simulink model "ControllerIntegration"  (R2020a)
settings: configuration reference "Configuration" (kept outside this file)
undefined symbols (not defined in the file or in its folder): Param
settings Model: Creator=12650014  LastModifiedBy=12650008
settings ConfigSetRef: SourceName=Configuration  SourceLocation=Base Workspace

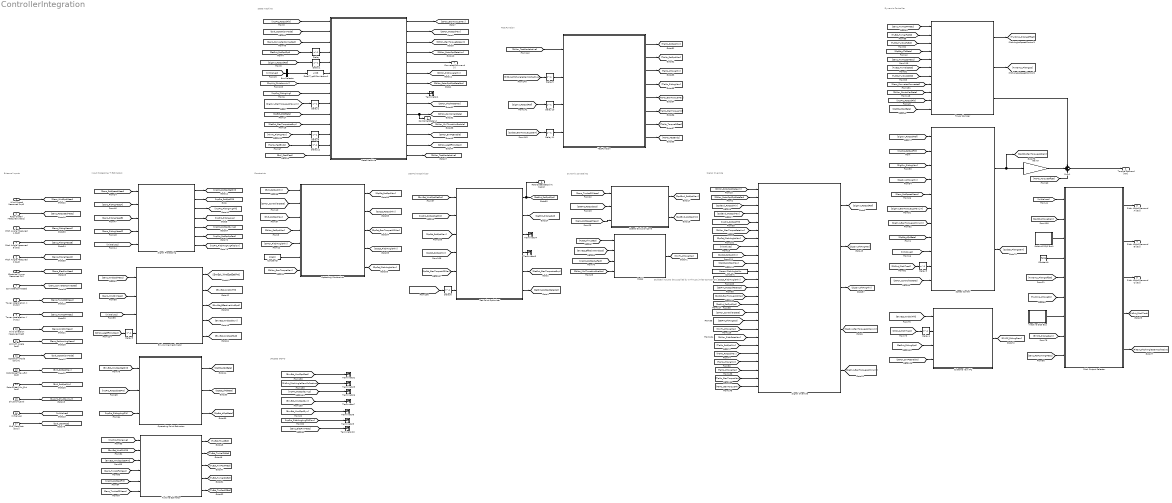
== system ControllerIntegration ==
  note: Stubbed input to be supplied by a Thrust Limiter Component
  note: UNUSED GOTO
  note: Dynamic constraints
  note: Set Point Optimizer
  note: Signal Override
  note: State machine
  note: Constraints
  note: Dynamic Controller
  note: Input Processing + Estimators
  note: External inputs
  note: Test Function
  Wind Speed Measured [m/s] : Inport
  Rotor Speed Measured [rad/s] : Inport  Port=2
  Pitch Angle Measured A [rad] : Inport  Port=3
  Pitch Angle Measured B [rad] : Inport  Port=4
  Pitch Angle Measured C [rad] : Inport  Port=5
  Electrical Power Measured [W] : Inport  Port=6
  ConverterConnected : Inport  Port=7
  Tower Acceleration X [m/s2] : Inport  Port=8
  Tower Acceleration Y [m/s2] : Inport  Port=9
  Wind Direction Measured [rad] : Inport  Port=10
  Azimuth Angle [rad] : Inport  Port=11
  Operation Mode [enum] : Inport  Port=12  OutDataTypeStr=Enum: OpMode
  RotorSpeedMax_Ext [rad] : Inport  Port=13
  RotorSpeedMin_Ext [rad] : Inport  Port=14
  ShudownLevel : Inport  Port=15
  InitValues : Inport  Port=16  OutDataTypeStr=Bus: InitVals
  Extl_StartTest [bool] : Inport  Port=17  OutDataTypeStr=boolean
  Bus Selector : BusSelector  OutputSignals=ControllerState
  Constant : Constant  Value=Param.PitchAngleMin
  Constant1 : Constant  Value=false
  Constant3 : Constant  Value=10e10
  Data Type Conversion1 : DataTypeConversion  OutDataTypeStr=uint8  RndMeth=Round
  Delay{,1..6,8..12} (12 alike) : Delay  DelayLength=1  InitialCondition=0
  Environment estimator : ModelReference  ModelNameDialog=EnvironmentEstimator.slx  SimulationMode=Normal  ModelReferenceVersion=1.228
  Extreme Yaw IPC : ModelReference  ModelNameDialog=ExtremeYawIPC.slx  SimulationMode=Normal  ModelReferenceVersion=1.200
  Gain9 : Gain  Gain=1/Param.GearRatio
  Inactive DQ0 Bus : Subsystem
  Inactive DQ0 Bus1 : Subsystem
  Model : ModelReference  ModelNameDialog=MinimumThrustLimiter.slx  SimulationMode=Normal  ModelReferenceVersion=1.237
  Operating Constraints : ModelReference  ModelNameDialog=OperatingConstraints.slx  SimulationMode=Normal  ModelReferenceVersion=1.199
  Operating Point Estimator : ModelReference  ModelNameDialog=OperatingPointEstimator.slx  SimulationMode=Normal  ModelReferenceVersion=1.187
  Pitch Output Selector : ModelReference  ModelNameDialog=PitchOutputSelector.slx  SimulationMode=Normal  ModelReferenceVersion=1.211
  Set Point Optimizer : ModelReference  ModelNameDialog=SetPointOptimizer.slx  SimulationMode=Normal  ModelReferenceVersion=1.164
  Signal Override : ModelReference  ModelNameDialog=SignalOverride.slx  SimulationMode=Normal  ModelReferenceVersion=1.219
  Signal Processing : ModelReference  ModelNameDialog=SignalProcessing.slx  SimulationMode=Normal  ModelReferenceVersion=1.117
  Speed Control : ModelReference  ModelNameDialog=SpeedController.slx  SimulationMode=Normal  ModelReferenceVersion=1.218
      settings: PortSchema="{\"entries\":[{\"content\":{\"sides\":[{\"content\":{\"connectorIds\":[\"In1\",\"In2\",\"In3\",\"In4\",\"In9\",\"In5\",\"In6\",\"In8\",\"In7\",\"In10\",\"In11\"]},\"type\":\"ConnectorPlacement.EquallySpacedRectSide\",\"uuid\":\"0d9f98d5-5863-4158-b9d8-c1cd92811ae6\"},{\"content\":{\"connectorIds\":[\"Out1\",\"Out2\"],\"side\":\"RIGHT\"},\"type\":\"ConnectorPlacement.EquallySpacedRectSide\",\"uuid\":\"8166d279-4671-4a5d-9b5c-a0ddc413a77e\"},{\"content\":{\"connectorIds\":[],\"side\":\"TOP\"},\"type\":\"ConnectorPlacement.EquallySpacedRectSide\",\"uuid\":\"e681da18-f7d9-4182-9560-dcdd8831121b\"}]},\"type\":\"ConnectorPlacement.EquallySpacedConnector\",\"uuid\":\"20163037-d862-4ea8-8a87-0fce0e65d82b\"}],\"packageUris\":[\"http://schema.mathworks.com/mf0/Connector/19700101\"],\"version\":\"1.0\"}"
  Speed ExclusionZone : ModelReference  ModelNameDialog=SpeedExclusionZone.slx  SimulationMode=Normal  ModelReferenceVersion=1.224
  State Machine : ModelReference  ModelNameDialog=StateMachine.slx  SimulationMode=Normal  ModelReferenceVersion=1.330
  Sum1 : Sum  Inputs=+++
  Terminator{1..10} (10 alike) : Terminator
  TestFunction : ModelReference  ModelNameDialog=TestMode.slx  SimulationMode=Normal  ModelReferenceVersion=1.381
  Tower damper : ModelReference  ModelNameDialog=TowerDamping.slx  SimulationMode=Normal  ModelReferenceVersion=1.225
  Turbine Estimator : ModelReference  ModelNameDialog=TurbineEstimator.slx  SimulationMode=Normal  ModelReferenceVersion=1.224
  ControllerState [-] : Outport  OutDataTypeStr=Enum: ControllerState
  Torque Demand [Nm] : Outport  Port=2
  Pitch Angle Demand A [rad] : Outport  Port=3
  Pitch Angle Demand B [rad] : Outport  Port=4
  Pitch Angle Demand C [rad] : Outport  Port=5
  RotorSpeedSetpoint [rad/s] : Outport  Port=6
  ConverterCommand [-] : Outport  Port=7
  wires:
  Wind Speed Measured [m/s]/1 -> [Sens_WndSpdMeas]
  Rotor Speed Measured [rad/s]/1 -> [Sens_RotSpeedMeas]
  [Sens_ConverterConnected] -> State Machine/3
  Signal Processing/2 -> [InpPrc_RotSpdFilt]
  [InpPrc_RotSpdFilt] -> Speed Control/2
  [InpPrc_RotSpdFilt] -> State Machine/1
  Delay/1 -> State Machine/4
  Delay1/1 -> State Machine/5
  [SetPnt_RotSpdOpt] -> Delay/1
  [SigOvr_RotSpdRef] -> Delay1/1
  Set Point Optimizer/6 -> [SetPnt_RotSpdRateOpt]
  Signal Processing/4 -> [InpPrc_PitAngAvg]
  [InpPrc_PitAngAvg] -> State Machine/8
  [SigOvr_GenTorqueLssMaxLim] -> Delay2/1
  State Machine/1 -> [StMcn_GenTorqueMax]
  State Machine/2 -> [StMcn_RotSpdMax]
  State Machine/3 -> [StMcn_GenTorqueRateLim]
  State Machine/4 -> [StMcn_RotorSpdRateLim]
  State Machine/5 -> ConverterCommand [-]/1
  [StMcn_RotorSpdRateLim] -> Signal Override/1
  [StMcn_GenTorqueMax] -> Operating Constraints/7
  State Machine/6 -> [StMcn_PitchAngleMin]
  Delay2/1 -> State Machine/9
  [InpPrc_RotSpdSetPnt] -> Set Point Optimizer/2
  [InitValues] -> Signal Processing/5
  Operating Point Estimator/1 -> [OpEst_dQdBeta]
  [StMcn_RotorSpdOptRateFac] -> Signal Override/2
  State Machine/7 -> [StMcn_RotorSpdOptRateFac]
  [OpEst_dQdBeta] -> State Machine/10
  [SetPnt_GenTorqueLssExp] -> State Machine/11
  [Extl_OperationMode] -> State Machine/2
  InitValues/1 -> [InitValues]
  Tower damper/1 -> [TwrDmp_PitAngOffset]
  Tower Acceleration X [m/s2]/1 -> [Sens_TwrAccSSMeas]
  [Sens_TwrAccSSMeas] -> Speed ExclusionZone/1
  [Sens_RotSpeedMeas] -> Speed ExclusionZone/3
  Speed ExclusionZone/1 -> [SpdExcl_RotSpdMax]
  Speed ExclusionZone/2 -> [SpdExcl_RotSpdMin]
  [SetPnt_RotSpdOpt] -> Speed ExclusionZone/2
  ShudownLevel/1 -> [SupVis_ShutdownLvl]
  Tower Acceleration Y [m/s2]/1 -> [Sens_TwrAccFAMeas]
  [TuEst_TwrVelFAEst] -> Tower damper/2
  Wind Direction Measured [rad]/1 -> [Sens_WndDirMeas]
  Set Point Optimizer/2 -> [SetPnt_PitAngOpt]
  Sum1/1 -> Torque Demand [Nm]/1
  Electrical Power Measured [W]/1 -> [Sens_ElecPwrMeas]
  RotorSpeedMax_Ext [rad]/1 -> [Extl_RotSpdMax]
  RotorSpeedMin_Ext [rad]/1 -> [Extl_RotSpdMin]
  [SpdExcl_RotSpdMin] -> Signal Override/3
  [SpdExcl_RotSpdMax] -> Signal Override/4
  State Machine/8 -> Terminator1/1
  [TuEst_TwrPosFAEst] -> Tower damper/3
  [OpEst_dTdBeta] -> Tower damper/4
  Operating Point Estimator/2 -> [OpEst_dTdBeta]
  Azimuth Angle [rad]/1 -> [Sens_RotAzmAngMeas]
  Pitch Angle Measured A [rad]/1 -> [Sens_PitAngMeasA]
  Pitch Angle Measured B [rad]/1 -> [Sens_PitAngMeasB]
  Pitch Angle Measured C [rad]/1 -> [Sens_PitAngMeasC]
  ConverterConnected/1 -> [Sens_ConverterConnected]
  Operation Mode [enum]/1 -> [Extl_OperationMode]
  [SupVis_ShutdownLvl] -> State Machine/7
  State Machine/9 -> [StMcn_PitchRateMax]
  [Sens_PitAngMeasC] -> Signal Processing/4
  [Sens_PitAngMeasB] -> Signal Processing/3
  [Sens_PitAngMeasA] -> Signal Processing/2
  [Sens_RotSpeedMeas] -> Signal Processing/1
  Signal Processing/1 -> [InpPrc_RotSpdSetPnt]
  Signal Processing/3 -> [InpPrc_PitAngAvgFilt]
  [Sens_TwrAccFAMeas] -> Tower damper/1
  [Sens_WndSpdMeas] -> Environment estimator/1
  [InpPrc_PitAngAvgFilt] -> Operating Point Estimator/3
  Turbine Estimator/1 -> [TuEst_ThrustEst]
  Turbine Estimator/2 -> [TuEst_TwrVelFAEst]
  Turbine Estimator/3 -> [TuEst_TwrPosFAEst]
  Turbine Estimator/5 -> [TuEst_TwrPosSSEst]
  Turbine Estimator/4 -> [TuEst_TwrVelSSEst]
  Pitch Output Selector/3 -> Pitch Angle Demand C [rad]/1
  Pitch Output Selector/2 -> Pitch Angle Demand B [rad]/1
  Pitch Output Selector/1 -> Pitch Angle Demand A [rad]/1
  Signal Override/2 -> [SigOvr_PitAngMax]
  Signal Override/3 -> [SigOvr_PitAngMin]
  Signal Override/4 -> [SigOvr_GenTorqueLssMaxLim]
  [SigOvr_GenTorqueLssMaxLim] -> Speed Control/5
  [SigOvr_GenTorqueLssMinLim] -> Speed Control/6
  [SigOvr_PitAngMin] -> Speed Control/4
  [SigOvr_PitAngMax] -> Speed Control/3
  [SigOvr_RotSpdRef] -> Speed Control/1
  Signal Override/1 -> [SigOvr_RotSpdRef]
  [Extl_RotSpdMin] -> Operating Constraints/1
  [Extl_RotSpdMax] -> Operating Constraints/3
  [StMcn_RotSpdMax] -> Operating Constraints/4
  [EnvEst_WndSpdSetPnt] -> Set Point Optimizer/1
  [StMcn_ControllerState] -> Operating Constraints/2
  Set Point Optimizer/5 -> [SetPnt_GenTorqueLssExp]
  State Machine/10 -> [StMcn_ControllerState], ControllerState [-]/1
  Operating Constraints/5 -> [OpCst_PitchAngleMax]
  Operating Constraints/4 -> [OpCst_PitchAngleMin]
  [SigOvr_GenTorqueLssMinLim] -> Delay6/1
  Operating Constraints/1 -> [OpCst_RotSpdMax]
  Operating Constraints/2 -> [OpCst_RotSpdMin]
  Operating Constraints/3 -> [OpCst_GenTorqueLSSMax]
  [OpCst_GenTorqueLSSMax] -> Set Point Optimizer/5
  [OpCst_RotSpdMin] -> Set Point Optimizer/4
  [OpCst_RotSpdMax] -> Set Point Optimizer/3
  Set Point Optimizer/1 -> [SetPnt_RotSpdOpt], RotorSpeedSetpoint [rad/s]/1
  Signal Override/5 -> [SigOvr_GenTorqueLssMinLim]
  [InpPrc_RotSpdFilt] -> Signal Override/5
  Bus Selector/1 -> Data Type Conversion1/1  "<ControllerState>"
  [InitValues] -> Bus Selector/1
  Data Type Conversion1/1 -> State Machine/6
  Set Point Optimizer/3 -> Terminator4/1
  Set Point Optimizer/4 -> Terminator3/1
  Speed Control/1 -> [SpdCtr_GenTorqueLssDem], Gain9/1
  Gain9/1 -> Sum1/2
  Delay6/1 -> Set Point Optimizer/6
  State Machine/11 -> [StMcn_MinThrustLimEnable]
  State Machine/12 -> [StMcn_EYIPCEnable]
  State Machine/13 -> [StMcn_UseEffWndSpd]
  [StMcn_MinThrustLimEnable] -> Model/4
  [TuEst_ThrustEst] -> Model/1
  [EnvEst_EffectiveWndSpd] -> Model/2
  Signal Processing/5 -> [InpPrc_RotSpdDynLp]
  Signal Processing/6 -> [InpPrc_RotSpdLpFast]
  [InpPrc_RotSpdLpFast] -> Model/3
  Model/1 -> [MinTL_PitAngMax]
  [EnvEst_WndDirFilt] -> Extreme Yaw IPC/1
  Extreme Yaw IPC/1 -> [EYIPC_PitAngDem]
  [SetPnt_PitAngOpt] -> Extreme Yaw IPC/3
  [StMcn_EYIPCEnable] -> Extreme Yaw IPC/4
  Speed Control/2 -> [SpdCtr_PitAngDem]
  [PitOut_PitchTrack] -> Delay4/1
  Delay4/1 -> Extreme Yaw IPC/2
  Constant3/1 -> Operating Constraints/6
  [StMcn_PitchAngleMin] -> Operating Constraints/5
  [EnvEst_WndSpdFast] -> Terminator2/1
  [StMcn_UseEffWndSpd] -> Delay5/1
  Delay5/1 -> Environment estimator/4
  [MinTL_PitAngMax] -> Signal Override/18
  [SetPnt_PitAngOpt] -> Signal Override/17
  [StMcn_ControllerState] -> Signal Override/16
  [SetPnt_RotSpdOpt] -> Signal Override/15
  [OpCst_GenTorqueLSSMax] -> Signal Override/14
  [SetPnt_RotSpdRateOpt] -> Signal Override/13
  [OpCst_PitchAngleMin] -> Signal Override/12
  Constant/1 -> Signal Override/11
  [OpCst_RotSpdMax] -> Signal Override/10
  [OpCst_RotSpdMin] -> Signal Override/9
  [InitValues] -> Signal Override/8
  [OpCst_PitchAngleMax] -> Signal Override/7
  [StMcn_GenTorqueRateLim] -> Signal Override/6
  [Sens_RotSpeedMeas] -> Speed Control/9
  Pitch Output Selector/4 -> [PitOut_PitchTrack]
  [InitValues] -> Pitch Output Selector/1
  [SpdCtr_PitAngDem] -> Pitch Output Selector/2
  Inactive DQ0 Bus1/1(DQ0 inactive) -> Pitch Output Selector/3
  Constant1/1 -> Pitch Output Selector/4
  [TwrDmp_PitAngOffset] -> Pitch Output Selector/5
  [TwrDmp_PitAngSS] -> Pitch Output Selector/6
  Inactive DQ0 Bus/1(DQ0 inactive) -> Pitch Output Selector/7
  [EYIPC_PitAngDem] -> Pitch Output Selector/8
  [Sens_RotAzmAngMeas] -> Pitch Output Selector/9
  [StMcn_PitchRateMax] -> Signal Override/19
  [Sens_TwrAccSSMeas] -> Turbine Estimator/6
  [InpPrc_PitAngAvg] -> Turbine Estimator/1
  [EnvEst_WndDirFilt] -> Turbine Estimator/2
  [EnvEst_WndSpdSetPnt] -> Turbine Estimator/3
  [Sens_TwrAccFAMeas] -> Turbine Estimator/4
  [InpPrc_RotSpdFilt] -> Turbine Estimator/5
  [TuEst_TwrPosSSEst] -> Tower damper/7
  [TuEst_TwrVelSSEst] -> Tower damper/6
  [Sens_TwrAccSSMeas] -> Tower damper/5
  Pitch Output Selector/5 -> [PitOut_PitchAngleDemCollective]
  Signal Processing/7 -> [InpPrc_PitchAngAvgFiltSlow]
  [PitOut_PitchAngleDemCollective] -> Terminator5/1
  [InpPrc_RotSpdDynLp] -> Terminator6/1
  [EnvEst_WndSpdDyn] -> Terminator7/1
  Delay8/1 -> State Machine/12
  [MinTL_PitAngMax] -> Delay8/1
  [EnvEst_WndSpdDyn] -> Terminator8/1
  [InpPrc_PitchAngAvgFiltSlow] -> Terminator9/1
  [Sens_WndDirMeas] -> Environment estimator/2
  Environment estimator/1 -> [EnvEst_WndSpdSetPnt]
  Environment estimator/2 -> [EnvEst_WndDirFilt]
  Environment estimator/3 -> [EnvEst_EffectiveWndSpd]
  Environment estimator/4 -> [EnvEst_WndSpdDyn]
  Environment estimator/5 -> [EnvEst_WndSpdFast]
  [InitValues] -> Environment estimator/3
  [EnvEst_WndSpdSetPnt] -> Operating Point Estimator/1
  [InpPrc_RotSpdSetPnt] -> Operating Point Estimator/2
  [Sens_ElecPwrMeas] -> Terminator10/1
  [PitOut_PitchTrack] -> Delay3/1
  Delay3/1 -> Speed Control/10
  [InitValues] -> Speed Control/7
  [OpEst_dQdBeta] -> Speed Control/8
  [StMcn_ControllerState] -> Tower damper/9
  [Sens_ConverterConnected] -> Tower damper/8
  [StMcn_ControllerState] -> Speed Control/11
  [TeMo_TestEnds] -> Delay12/1
  Delay12/1 -> State Machine/13
  Delay11/1 -> TestFunction/4
  [SpdCtr_GenTorqueLssDem] -> Delay11/1
  Delay10/1 -> TestFunction/3
  [SigOvr_RotSpdRef] -> Delay10/1
  Delay9/1 -> TestFunction/2
  [PitOut_PitchAngleDemCollective] -> Delay9/1
  [StMcn_TestModeActive] -> TestFunction/1
  State Machine/14 -> [StMcn_TestModeActive]
  TestFunction/8 -> [TeMo_TestEnds]
  TestFunction/7 -> [TeMo_TorqueOffset]
  TestFunction/6 -> [TeMo_GenTorqueMin]
  TestFunction/2 -> [TeMo_RotSpdMax]
  TestFunction/3 -> [TeMo_PitAngMin]
  TestFunction/5 -> [TeMo_GenTorqueMax]
  TestFunction/4 -> [TeMo_PitAngMax]
  TestFunction/1 -> [TeMo_RotSpdMin]
  [TeMo_RotSpdMax] -> Signal Override/21
  [TeMo_PitAngMax] -> Signal Override/23
  [TeMo_GenTorqueMin] -> Signal Override/25
  [TeMo_PitAngMin] -> Signal Override/22
  [TeMo_GenTorqueMax] -> Signal Override/24
  [TeMo_RotSpdMin] -> Signal Override/20
  Extl_StartTest [bool]/1 -> [Extl_StartTest]
  [Extl_StartTest] -> State Machine/14
  Operating Point Estimator/3 -> [OpEst_dCqdBeta]
  [InpPrc_RotSpdFilt] -> Tower damper/10
  [OpEst_dCqdBeta] -> Tower damper/11
  Tower damper/3 -> Sum1/1
  Tower damper/2 -> [TwrDmp_PitAngSS]
  [TeMo_TorqueOffset] -> Sum1/3

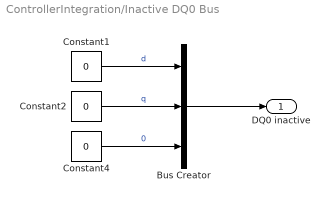
== system ControllerIntegration/Inactive DQ0 Bus ==
  Bus Creator : BusCreator  Inputs=3  OutDataTypeStr=Bus: Dq0Bus
      settings: InheritFromInputs=off
  Constant1 : Constant  Value=0
  Constant2 : Constant  Value=0
  Constant4 : Constant  Value=0
  DQ0 inactive : Outport
  wires:
  Constant1/1 -> Bus Creator/1  "d"
  Constant2/1 -> Bus Creator/2  "q"
  Bus Creator/1 -> DQ0 inactive/1
  Constant4/1 -> Bus Creator/3  "0"

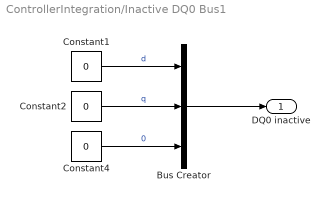
== system ControllerIntegration/Inactive DQ0 Bus1 ==
  Bus Creator : BusCreator  Inputs=3  OutDataTypeStr=Bus: Dq0Bus
      settings: InheritFromInputs=off
  Constant1 : Constant  Value=0
  Constant2 : Constant  Value=0
  Constant4 : Constant  Value=0
  DQ0 inactive : Outport
  wires:
  Constant1/1 -> Bus Creator/1  "d"
  Constant2/1 -> Bus Creator/2  "q"
  Bus Creator/1 -> DQ0 inactive/1
  Constant4/1 -> Bus Creator/3  "0"
